simulink model "HapticController"  (R2018a)
settings: Solver=ode23s  StartTime=0.0  StopTime=7  MaxStep=0.001
values from neighbouring files (symbols this model uses):
  B_e = 50    [HapticsSetup.m]
  K_e = 100000    [HapticsSetup.m]
  m = 1    [HapticsSetup.m]
undefined symbols (not defined in the file or in its folder): getCollision, K_p
libraries: simulink x1
settings Model: Creator=augus  LastModifiedBy=augus

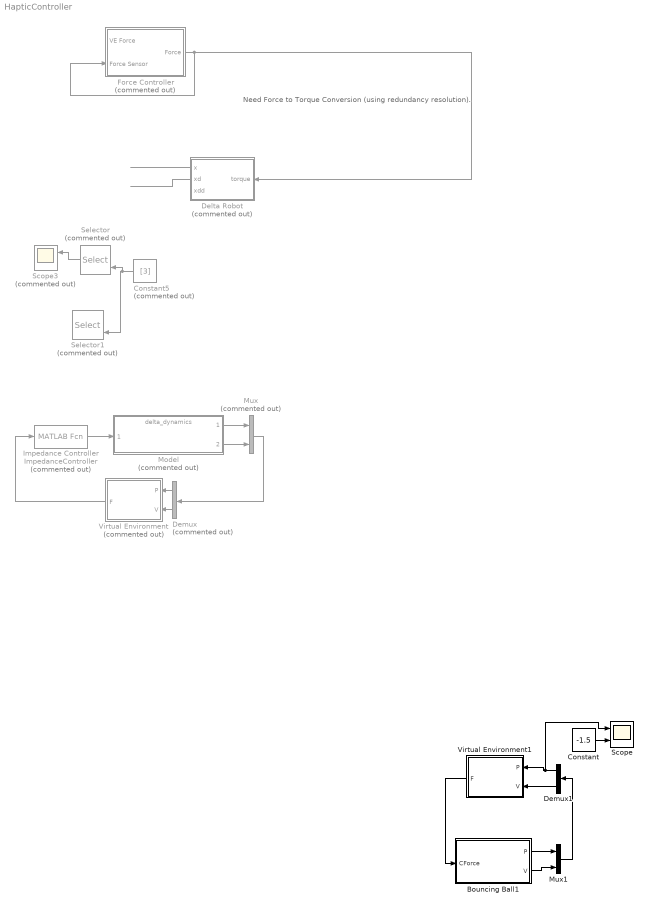
== system HapticController ==
  note: Need Force to Torque Conversion (using redundancy resolution).
  Bouncing Ball1 : Subsystem
  Constant : Constant  Value=-1.5
  Constant5 : Constant  Commented=on  Value=[3]
  Delta Robot : Subsystem  Commented=on
  Demux : Demux  Commented=on  Outputs=2
  Demux1 : Demux  Outputs=2
  Force Controller : Subsystem  Commented=on
  "Impedance Controller " : MATLABFcn  Commented=on  MATLABFcn=ImpedanceController
  Model : ModelReference  Commented=on  ModelNameDialog=delta_dynamics  SimulationMode=Normal  ModelReferenceVersion=1.9
  Mux : Mux  Commented=on  Inputs=2
  Mux1 : Mux  Inputs=2
  Scope : Scope  NumInputPorts=2
  Scope3 : Scope  Commented=on  NumInputPorts=2
  Selector : Selector  Commented=on  InputPortWidth=6  IndexOptions=Index vector (port)  Indices=[1 3]  OutputSizes=1
  Selector1 : Selector  Commented=on  InputPortWidth=6  IndexOptions=Index vector (port)  Indices=[1 3]  OutputSizes=1
  Virtual Environment : Subsystem  Commented=on
  Virtual Environment1 : Subsystem
  wires:
  Delta Robot/1(x) -> ?
  Delta Robot/2(xd) -> ?
  ? -> Force Controller/1(VE Force)
  Force Controller/1(Force) -> Force Controller/2(Force Sensor), Delta Robot/1("torque ")
  Constant5/1 -> Selector1/2, Selector/2
  Demux/2 -> Virtual Environment/2(V)
  Demux/1 -> Virtual Environment/1(P)
  Selector/1 -> Scope3/1
  Model/1 -> Mux/1
  Model/2 -> Mux/2
  Mux/1 -> Demux/1
  Demux1/2 -> Virtual Environment1/2(V)
  Demux1/1 -> Scope/1, Virtual Environment1/1(P)
  Bouncing Ball1/1(P) -> Mux1/1
  Bouncing Ball1/2(V) -> Mux1/2
  Mux1/1 -> Demux1/1
  Virtual Environment1/1(F) -> Bouncing Ball1/1(CForce)
  "Impedance Controller "/1 -> Model/1
  Virtual Environment/1(F) -> "Impedance Controller "/1
  Constant/1 -> Scope/2

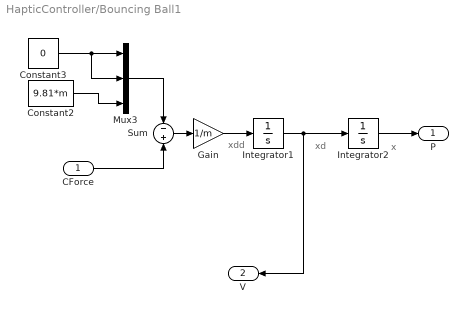
== system HapticController/Bouncing Ball1 ==
  note: xdd
  note: xd
  note: x
  CForce : Inport
  Constant2 : Constant  Value=9.81*m
  Constant3 : Constant  Value=0
  Gain : Gain  Gain=1/m
  Integrator1 : Integrator  InitialCondition=[0;0;0]
  Integrator2 : Integrator  InitialCondition=[0;0;-0.5]
  Mux3 : Mux  Inputs=3
  Sum : Sum  Inputs=-+
  P : Outport
  V : Outport  Port=2
  wires:
  Integrator1/1 -> V/1, Integrator2/1
  Gain/1 -> Integrator1/1
  Sum/1 -> Gain/1
  Constant2/1 -> Mux3/3
  Constant3/1 -> Mux3/1, Mux3/2
  Mux3/1 -> Sum/1
  Integrator2/1 -> P/1
  CForce/1 -> Sum/2

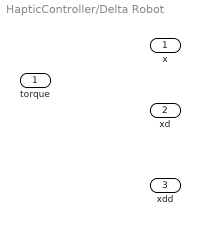
== system HapticController/Delta Robot ==
  "torque " : Inport
  x : Outport
  xd : Outport  Port=2
  xdd : Outport  Port=3

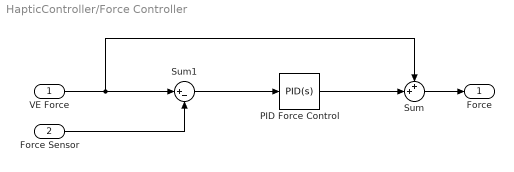
== system HapticController/Force Controller ==
  VE Force : Inport
  Force Sensor : Inport  Port=2
  "PID Force Control " : simulink/Continuous/PID Controller  Controller=PID  TimeDomain=Continuous-time  SampleTime=-1  IntegratorMethod=Forward Euler  FilterMethod=Forward Euler  Form=Parallel  UseFilter=on  ControllerParametersSource=internal  P=K_p  I=1  D=0  N=100  InitialConditionSource=internal  InitialConditionForIntegrator=0  InitialConditionForFilter=0  ExternalReset=none  LimitOutput=off  UpperSaturationLimit=inf  LowerSaturationLimit=-inf  LinearizeAsGain=on  AntiWindupMode=none  Kb=1  TrackingMode=off  Kt=1  PParamMin=[]  PParamMax=[]  IParamMin=[]  IParamMax=[]  DParamMin=[]  DParamMax=[]  NParamMin=[]  NParamMax=[]  KbParamMin=[]  KbParamMax=[]  KtParamMin=[]  KtParamMax=[]  POutMin=[]  POutMax=[]  IOutMin=[]  IOutMax=[]  DOutMin=[]  DOutMax=[]  NOutMin=[]  NOutMax=[]  KbOutMin=[]  KbOutMax=[]  KtOutMin=[]  KtOutMax=[]  IntegratorOutMin=[]  IntegratorOutMax=[]  FilterOutMin=[]  FilterOutMax=[]  SumOutMin=[]  SumOutMax=[]  SumI1OutMin=[]  SumI1OutMax=[]  SumI2OutMin=[]  SumI2OutMax=[]  SumI3OutMin=[]  SumI3OutMax=[]  SumDOutMin=[]  SumDOutMax=[]  SaturationOutMin=[]  SaturationOutMax=[]  IntegratorContinuousStateAttributes=''  IntegratorStateMustResolveToSignalObject=off  IntegratorRTWStateStorageClass=Auto  FilterContinuousStateAttributes=''  FilterStateMustResolveToSignalObject=off  FilterRTWStateStorageClass=Auto  DifferentiatorICPrevScaledInput=0  DifferentiatorOutMin=[]  DifferentiatorOutMax=[]  FilterDiffOutCoefMin=[]  FilterDiffOutCoefMax=[]  SumDenOutMin=[]  SumDenOutMax=[]  SumNumOutMin=[]  SumNumOutMax=[]  ReciprocalOutMin=[]  ReciprocalOutMax=[]  DivideOutMin=[]  DivideOutMax=[]  TunerSelectOption=Transfer Function Based (PID Tuner App)
  Sum : Sum  Inputs=++|
  Sum1 : Sum  Inputs=|+-
  Force : Outport
  wires:
  Sum/1 -> Force/1
  Force Sensor/1 -> Sum1/2
  Sum1/1 -> "PID Force Control "/1
  VE Force/1 -> Sum/1, Sum1/1
  "PID Force Control "/1 -> Sum/2

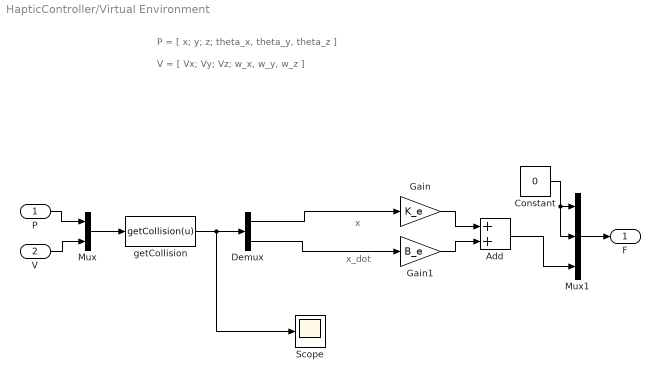
== system HapticController/Virtual Environment ==
  note: x_dot
  note: x
  note: P = [ x; y; z; theta_x, theta_y, theta_z ]
  note: V = [ Vx; Vy; Vz; w_x, w_y, w_z ]
  P : Inport
  V : Inport  Port=2
  Add : Sum
  Constant : Constant  Value=0
  Demux : Demux  Outputs=2
  Gain : Gain  Gain=K_e
  Gain1 : Gain  Gain=B_e
  Mux : Mux  Inputs=2
  Mux1 : Mux  Inputs=3
  Scope : Scope
  getCollision : MATLABFcn  MATLABFcn=getCollision(u)  OutputDimensions=2
  F : Outport
  wires:
  P/1 -> Mux/1
  V/1 -> Mux/2
  Gain/1 -> Add/1
  Gain1/1 -> Add/2
  Mux/1 -> getCollision/1
  getCollision/1 -> Scope/1, Demux/1
  Demux/1 -> Gain/1
  Demux/2 -> Gain1/1
  Mux1/1 -> F/1
  Add/1 -> Mux1/3
  Constant/1 -> Mux1/2, Mux1/1

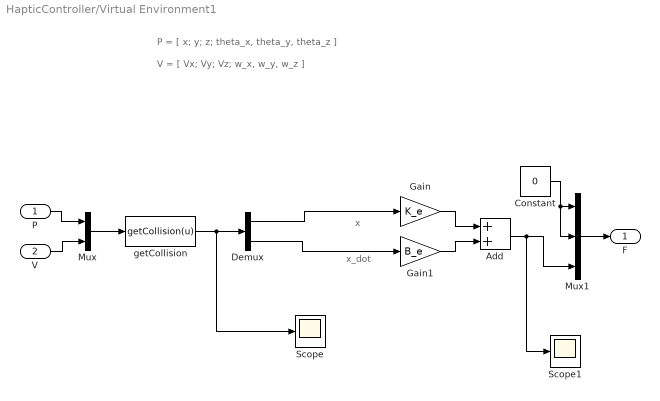
== system HapticController/Virtual Environment1 ==
  note: x_dot
  note: x
  note: P = [ x; y; z; theta_x, theta_y, theta_z ]
  note: V = [ Vx; Vy; Vz; w_x, w_y, w_z ]
  P : Inport
  V : Inport  Port=2
  Add : Sum
  Constant : Constant  Value=0
  Demux : Demux  Outputs=2
  Gain : Gain  Gain=K_e
  Gain1 : Gain  Gain=B_e
  Mux : Mux  Inputs=2
  Mux1 : Mux  Inputs=3
  Scope : Scope
  Scope1 : Scope
  getCollision : MATLABFcn  MATLABFcn=getCollision(u)  OutputDimensions=2
  F : Outport
  wires:
  P/1 -> Mux/1
  V/1 -> Mux/2
  Gain/1 -> Add/1
  Gain1/1 -> Add/2
  Mux/1 -> getCollision/1
  getCollision/1 -> Scope/1, Demux/1
  Demux/1 -> Gain/1
  Demux/2 -> Gain1/1
  Mux1/1 -> F/1
  Add/1 -> Scope1/1, Mux1/3
  Constant/1 -> Mux1/2, Mux1/1
